simulink model "w3_warplab_trigger_proc"  (Simulink 7.7)
settings: Solver=ode45  StartTime=0.0  StopTime=60  RelTol=1e-3
InitFcn:
  | w3_warplab_trigger_proc_init
StartFcn:
  | w3_warplab_trigger_proc_init
undefined symbols (not defined in the file or in its folder): gcbh, xlBlockLoadCallback, xlGetNormalizedPeriod
libraries: xbsIndex_r4 x1289, xbsEDKLib_r4 x1, simulink x1
(part 1 of 10)
settings Model: Creator=murphpo  LastModifiedBy=mango
settings DebuggingCC: FcnCallInpInsideContextMsg=Enable All

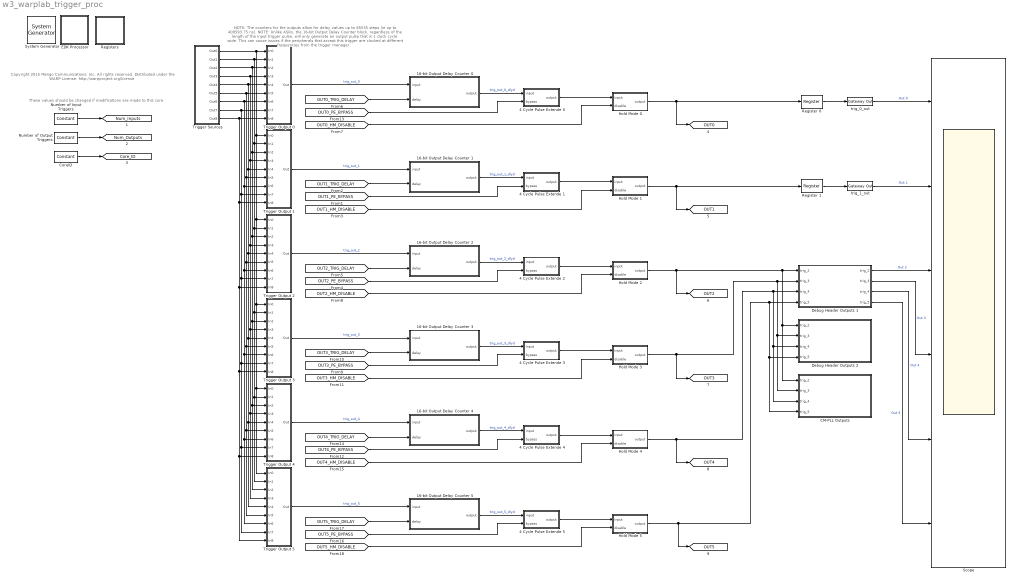
== system w3_warplab_trigger_proc ==
  note: These values should be changed if modifications are made to this core
  note: Copyright 2015 Mango Communications, Inc. All rights reserved.
      |
      | Distributed under the WARP License:
      | http://warpproject.org/license
  note: NOTE:  The counters for the outputs allow for delay values up to 65535 steps (ie up to 409593.75 ns).
      |
      | NOTE:  Unlike ASRs, the 16-bit Output Delay Counter block, regardless of the length of the input trigger
      | pulse, will only generate an output pulse that is 1 clock cycle wide. This can cause issues if the peripherals
      | that accept this trigger are clocked at different frequencies from the trigger manager.
  " System Generator" : xbsIndex_r4/ System Generator  Tag=genX  SystemSampleTime=-1  xilinxfamily=virtex6  part=xc6vlx240t  speed=-2  package=ff1156  synthesis_tool=XST  clock_wrapper=Clock Enables  directory=./trigger_proc  proj_type=Project Navigator  Synth_file=XST Defaults  Impl_file=ISE Defaults  testbench=off  simulink_period=1  sysclk_period=10  dcm_input_clock_period=10  incr_netlist=off  trim_vbits=Everywhere in SubSystem  dbl_ovrd=According to Block Masks  core_generation=According to Block Masks  run_coregen=off  deprecated_control=off  eval_field=0  block_type=sysgen
  16-bit Output Delay Counter 0 : Subsystem
  16-bit Output Delay Counter 1 : Subsystem
  16-bit Output Delay Counter 2 : Subsystem
  16-bit Output Delay Counter 3 : Subsystem
  16-bit Output Delay Counter 4 : Subsystem
  16-bit Output Delay Counter 5 : Subsystem
  4 Cycle Pulse Extende 0 : Subsystem
  4 Cycle Pulse Extende 1 : Subsystem
  4 Cycle Pulse Extende 2 : Subsystem
  4 Cycle Pulse Extende 3 : Subsystem
  4 Cycle Pulse Extende 4 : Subsystem
  4 Cycle Pulse Extende 5 : Subsystem
  CM-PLL Outputs : Subsystem
  CoreID : xbsIndex_r4/Constant  const=0  gui_display_data_type=Fixed-point  arith_type=Unsigned  n_bits=8  bin_pt=0  preci_type=Single  exp_width=8  frac_width=24  explicit_period=on  period=1  equ=P=C  opselect=C  inp2=PCIN>>17  opr=+  inp1=P  carry=CIN  dbl_ovrd=off  block_type=constant
  Debug Header Outputs 1 : Subsystem
  Debug Header Outputs 2 : Subsystem
  EDK Processor : Subsystem  LoadFcn=xlBlockLoadCallback(gcbh);  mask(Xilinx EDK Processor Block){mode=EDK pcore generation, xmp=, MemVisToProc=<qt bgcolor="#FFFFFF"><div><img src="C:/Xilinx/14.4/ISE_DS/ISE/sysgen/data/images/registerplus.gif"> &lt;&lt;TRIG_ODELAY_CFG_CMPLL&gt;&gt;<br></div><div><img src="C:/Xilinx/14.4/ISE_DS/ISE/sysgen/data/images/registerplus.gif"> &lt;&lt;TRIG_IDELAY_CFG_CMPLL&gt;&gt;<br></div><div><img src="C:/Xilinx/14.4/ISE_DS/ISE/sysgen/data/images/registerplus.gif"> &lt;&lt;TRIG_ODELAY_CFG_DEBUG_HDR&gt;&gt;<br></div><div><img src="C:/Xilinx/14.4/ISE_DS/ISE/sysgen/data/images/registerplus.gif"> &lt;&lt;TRIG_IDELAY_CFG_DEBUG_HDR&gt;&gt;<br></div><div><img src="C:/Xilinx/14.4/ISE_DS/ISE/sysgen/data/images/registerplus.gif"> &lt;&lt;TRIG_IODELAYS_CONTROL&gt;&gt;<br></div><div><img src="C:/Xilinx/14.4/ISE_DS/ISE/sysgen/data/images/registerplus.gif"> &lt;&lt;RSSI_PKT_DET_CONFIG&gt;&gt;<br></div><div><img src="C:/Xilinx/14.4/ISE_DS/ISE/sysgen/data/images/registerplus.gif"> &lt;&lt;TRIG_IN_CONF_6&gt;&gt;<br></div><div><img src="C:/Xilinx/14.4/ISE_DS/ISE/sysgen/data/images/registerplus.gif"> &lt;&lt;TRIG_IN_CONF_5&gt;&gt;<br></div><div><img src="C:/Xilinx/14.4/ISE_DS/ISE/sysgen/data/images/registerplus.gif"> &lt;&lt;TRIG_IN_CONF_4&gt;&gt;<br></div><div><img src="C:/Xilinx/14.4/ISE_DS/ISE/sysgen/data/images/registerplus.gif"> &lt;&lt;TRIG_IN_CONF_3&gt;&gt;<br></div><div><img src="C:/Xilinx/14.4/ISE_DS/ISE/sysgen/data/images/registerplus.gif"> &lt;&lt;TRIG_IN_CONF_2&gt;&gt;<br></div><div><img src="C:/Xilinx/14.4/ISE_DS/ISE/sysgen/data/images/registerplus.gif"> &lt;&lt;TRIG_IN_CONF_0&gt;&gt;<br></div><div><img src="C:/Xilinx/14.4/ISE_DS/ISE/sysgen/data/images/registerplus.gif"> &lt;&lt;TRIG_IN_CONF_8&gt;&gt;<br></div><div><img src="C:/Xilinx/14.4/ISE_DS/ISE/sysgen/data/images/registerplus.gif"> &lt;&lt;TRIG_IN_CONF_7&gt;&gt;<br></div><div><img src="C:/Xilinx/14.4/ISE_DS/ISE/sysgen/data/images/registerplus.gif"> &lt;&lt;TRIG_OUT_5_CONF_0&gt;&gt;<br></div><div><img src="C:/Xilinx/14.4/ISE_DS/ISE/sysgen/data/images/registerplus.gif"> &lt;&lt;TRIG_OUT_5_CONF_1&gt;&gt;<br></div><div><img src="C:/Xilinx/14.4/ISE_DS/ISE/sysgen/data/images/registerplus.gif"> &lt;&lt;TRIG_OUT_4_CONF_0&gt;&gt;<br></div><div><img src="C:/Xilinx/14.4/ISE_DS/ISE/sysgen/data/images/registerplus.gif"> &lt;&lt;TRIG_OUT_0_CONF_0&gt;&gt;<br></div><div><img src="C:/Xilinx/14.4/ISE_DS/ISE/sysgen/data/images/registerplus.gif"> &lt;&lt;TRIG_OUT_4_CONF_1&gt;&gt;<br></div><div><img src="C:/Xilinx/14.4/ISE_DS/ISE/sysgen/data/images/registerplus.gif"> &lt;&lt;TRIG_OUT_3_CONF_0&gt;&gt;<br></div><div><img src="C:/Xilinx/14.4/ISE_DS/ISE/sysgen/data/images/registerplus.gif"> &lt;&lt;TRIG_OUT_3_CONF_1&gt;&gt;<br></div><div><img src="C:/Xilinx/14.4/ISE_DS/ISE/sysgen/data/images/registerplus.gif"> &lt;&lt;TRIG_OUT_2_CONF_0&gt;&gt;<br></div><div><img src="C:/Xilinx/14.4/ISE_DS/ISE/sysgen/data/images/registerplus.gif"> &lt;&lt;TRIG_OUT_2_CONF_1&gt;&gt;<br></div><div><img src="C:/Xilinx/14.4/ISE_DS/ISE/sysgen/data/images/registerplus.gif"> &lt;&lt;TRIG_OUT_1_CONF_0&gt;&gt;<br></div><div><img src="C:/Xilinx/14.4/ISE_DS/ISE/sysgen/data/images/registerplus.gif"> &lt;&lt;TRIG_OUT_1_CONF_1&gt;&gt;<br></div><div><img src="C:/Xilinx/14.4/ISE_DS/ISE/sysgen/data/images/registerplus.gif"> &lt;&lt;TRIG_OUT_0_CONF_1&gt;&gt;<br></div><div><img src="C:/Xilinx/14.4/ISE_DS/ISE/sysgen/data/images/registerplus.gif"> &lt;&lt;RSSI_PKT_DET_DURATIONS&gt;&gt;<br></div><div><img src="C:/Xilinx/14.4/ISE_DS/ISE/sysgen/data/images/registerplus.gif"> &lt;&lt;RSSI_PKT_DET_THRESHOLDS&gt;&gt;<br></div><div><img src="C:/Xilinx/14.4/ISE_DS/ISE/sysgen/data/images/registerplus.gif"> &lt;&lt;TRIG_IN_CONF_1&gt;&gt;<br></div><div><img src="C:/Xilinx/14.4/ISE_DS/ISE/sysgen/data/images/registerplus.gif"> &lt;&lt;CORE_INFO&gt;&gt;<br></div><div><img src="C:/Xilinx/14.4/ISE_DS/ISE/sysgen/data/images/registerplus.gif"> &lt;&lt;TRIG_OUT&gt;&gt;<br></div><div><img src="C:/Xilinx/14.4/ISE_DS/ISE/sysgen/data/images/memoryplus.gif"> &lt;&lt;PktOps1&gt;&gt;<br></div><div><img src="C:/Xilinx/14.4/ISE_DS/ISE/sysgen/data/images/memoryplus.gif"> &lt;&lt;PktTemplate1&gt;&gt;<br></div><div><img src="C:/Xilinx/14.4/ISE_DS/ISE/sysgen/data/images/memoryplus.gif"> &lt;&lt;PktOps0&gt;&gt;<br></div><div><img src="C:/Xilinx/14.4/ISE_DS/ISE/sysgen/data/images/memoryplus.gif"> &lt;&lt;PktTemplate0&gt;&gt;<br></div></qt>, AvailableMemories=<empty>, portInterfaceTable={'exposed'=>[],'portdir'=>[],'portname'=>[],'shortname'=>[]}, bus_type_sgadvanced=, bus_type=AXI, baseaddr=0x80000000, baseaddr_lock_sgadvanced=, baseaddr_lock=off, dual_clock_sgadvanced=, dual_clock=on, reg_readback_sgadvanced=, reg_readback=on, ucf_file=, inheritDeviceType_sgadvanced=, inheritDeviceType=off, elf_file=, codebug_sgadvanced=, codebug=on, clock_name=plb, internalPortList={}, resetPolarity=0, memxtable={'mladdr'=>[0.00000000000000000,1.00000000000000000,2.00000000000000000,3.00000000000000000,4.00000000000000000,5.00000000000000000,6.00000000000000000,7.00000000000000000,8.00000000000000000,9.00000000000000000,10.00000000000000000,11.00000000000000000,12.00000000000000000,13.00000000000000000,14.00000000000000000,15.00000000000000000,16.00000000000000000,17.00000000000000000,18.00000000000000000,19.00000000000000000,20.00000000000000000,21.00000000000000000,22.00000000000000000,23.00000000000000000,24.00000000000000000,25.00000000000000000,26.00000000000000000,27.00000000000000000,28.00000000000000000,0.00000000000000000,1.00000000000000000,-1.00000000000000000,-1.00000000000000000,-1.00000000000000000,-1.00000000000000000],'mlist'=>['w3_warplab_trigger_proc/Registers/Trig IODELAY Config/From Register28','w3_warplab_trigger_proc/Registers/Trig IODELAY Config/From Register27','w3_warplab_trigger_proc/Registers/Trig IODELAY Config/From Register26','w3_warplab_trigger_proc/Registers/Trig IODELAY Config/From Register25','w3_warplab_trigger_proc/Registers/Trig IODELAY Config/From Register1','w3_warplab_trigger_proc/Registers/From Register9','w3_warplab_trigger_proc/Registers/From Register8','w3_warplab_trigger_proc/Registers/From Register7','w3_warplab_trigger_proc/Registers/From Register6','w3_warplab_trigger_proc/Registers/From Register5','w3_warplab_trigger_proc/Registers/From Register4','w3_warplab_trigger_proc/Registers/From Register3','w3_warplab_trigger_proc/Registers/From Register24','w3_warplab_trigger_proc/Registers/From Register23','w3_warplab_trigger_proc/Registers/From Register22','w3_warplab_trigger_proc/Registers/From Register21','w3_warplab_trigger_proc/Registers/From Register20','w3_warplab_trigger_proc/Registers/From Register2','w3_warplab_trigger_proc/Registers/From Register19','w3_warplab_trigger_proc/Registers/From Register18','w3_warplab_trigger_proc/Registers/From Register17','w3_warplab_trigger_proc/Registers/From Register16','w3_warplab_trigger_proc/Registers/From Register15','w3_warplab_trigger_proc/Registers/From Register14','w3_warplab_trigger_proc/Registers/From Register13','w3_warplab_trigger_proc/Registers/From Register12','w3_warplab_trigger_proc/Registers/From Register11','w3_warplab_trigger_proc/Registers/From Register10','w3_warplab_trigger_proc/Registers/From Register1','w3_warplab_trigger_proc/Registers/To Register1','w3_warplab_trigger_proc/Registers/To Register','w3_warplab_trigger_proc/Trigger Sources/Ethernet B/Pkt Comp/Word Comp 1/Shared Memory2','w3_warplab_trigger_proc/Trigger Sources/Ethernet B/Pkt Comp/Word Comp 1/Shared Memory1','w3_warplab_trigger_proc/Trigger Sources/Ethernet A/Pkt Comp/Word Comp 0/Shared Memory2','w3_warplab_trigger_proc/Trigger Sources/Ethernet A/Pkt Comp/Word Comp 0/Shared Memory1'],'mlname'=>['\\'TRIG_ODELAY_CFG_CMPLL\\'','\\'TRIG_IDELAY_CFG_CMPLL\\'','\\'TRIG_ODELAY_CFG_DEBUG_HDR\\'','\\'TRIG_IDELAY_CFG_DEBUG_HDR\\'','\\'TRIG_IODELAYS_CONTROL\\'','\\'RSSI_PKT_DET_CONFIG\\'','\\'TRIG_IN_CONF_6\\'','\\'TRIG_IN_CONF_5\\'','\\'TRIG_IN_CONF_4\\'','\\'TRIG_IN_CONF_3\\'','\\'TRIG_IN_CONF_2\\'','\\'TRIG_IN_CONF_0\\'','\\'TRIG_IN_CONF_8\\'','\\'TRIG_IN_CONF_7\\'','\\'TRIG_OUT_5_CONF_0\\'','\\'TRIG_OUT_5_CONF_1\\'','\\'TRIG_OUT_4_CONF_0\\'','\\'TRIG_OUT_0_CONF_0\\'','\\'TRIG_OUT_4_CONF_1\\'','\\'TRIG_OUT_3_CONF_0\\'','\\'TRIG_OUT_3_CONF_1\\'','\\'TRIG_OUT_2_CONF_0\\'','\\'TRIG_OUT_2_CONF_1\\'','\\'TRIG_OUT_1_CONF_0\\'','\\'TRIG_OUT_1_CONF_1\\'','\\'TRIG_OUT_0_CONF_1\\'','\\'RSSI_PKT_DET_DURATIONS\\'','\\'RSSI_PKT_DET_THRESHOLDS\\'','\\'TRIG_IN_CONF_1\\'','\\'CORE_INFO\\'','\\'TRIG_OUT\\'','\\'PktOps1\\'','\\'PktTemplate1\\'','\\'PktOps0\\'','\\'PktTemplate0\\''],'mlstate'=>[0.00000000000000000,0.00000000000000000,0.00000000000000000,0.00000000000000000,0.00000000000000000,0.00000000000000000,0.00000000000000000,0.00000000000000000,0.00000000000000000,0.00000000000000000,0.00000000000000000,0.00000000000000000,0.00000000000000000,0.00000000000000000,0.00000000000000000,0.00000000000000000,0.00000000000000000,0.00000000000000000,0.00000000000000000,0.00000000000000000,0.00000000000000000,0.00000000000000000,0.00000000000000000,0.00000000000000000,0.00000000000000000,0.00000000000000000,0.00000000000000000,0.00000000000000000,0.00000000000000000,0.00000000000000000,0.00000000000000000,0.00000000000000000,0.00000000000000000,0.00000000000000000,0.00000000000000000]}, procinfo={}, memmapdirty=off, blockname=, xpsintstyle=default, has_advanced_control=0, sggui_pos=-1,-1,-1,-1, block_type=edkprocessor, block_version=2.7, sg_icon_stat=62,64,-1,-1,white,blue,0,07734,right,,[ ],[ ], sg_mask_display=|, sg_list_contents={'table'=>{'AvailableMemories'=>'popup(<empty>)'}}, sg_blockgui_xml=}
      mask sg_mask_display=|
      | fprintf('','COMMENT: begin icon graphics');
      | patch([0 62 62 0 0 ],[0 0 64 64 0 ],[0.77 0.82 0.91 ]);
      | plot([0 62 62 0 0 ],[0 0 64 64 0 ]);
      | patch([13.2 24.76 32.76 40.76 48.76 32.76 21.2 13.2 ],[40.88 40.88 48.88 40.88 48.88 48.88 48.88 40.88 ],[1 1 1 ]);
      | patch([21.2 32.76 24.76 13.2 21.2 ],[32.88 32.88 40.88 40.88 32.88 ],[0.931 0.946 0.973 ]);
      | patch([13.2 24.76 32.76 21.2 13.2 ],[24.88 24.88 32.88 32.88 24.88 ],[1 1 1 ]);
      | patch([21.2 48.76 40.76 32.76 24.76 13.2 21.2 ],[16.88 16.88 24.88 16.88 24.88 24.88 16.88 ],[0.931 0.946 0.973 ]);
      | fprintf('','COMMENT: end icon graphics');
      | fprintf('','COMMENT: begin icon text');
      | fprintf('','COMMENT: end icon text');
      mask prompts: mode "Configure Processor for"; xmp "XPS Project"; MemVisToProc ""; AvailableMemories "Available Memories"; portInterfaceTable ""; bus_type_sgadvanced ""; bus_type "Bus Type"; baseaddr "Base Address"; baseaddr_lock_sgadvanced ""; baseaddr_lock "Lock"; dual_clock_sgadvanced ""; dual_clock "Dual Clocks"; reg_readback_sgadvanced ""; reg_readback "Register Read-Back"; ucf_file "Constraint File"; inheritDeviceType_sgadvanced ""; inheritDeviceType "Inherit Device Type"; elf_file "Initial Program"; codebug_sgadvanced ""; codebug "Enable Co-Debug with Xilinx SDK (Beta)"; clock_name ""; internalPortList ""; resetPolarity ""; memxtable ""; procinfo ""; memmapdirty ""; blockname ""; xpsintstyle ""; has_advanced_control ""; sggui_pos ""; block_type ""; block_version ""; sg_icon_stat ""; sg_mask_display ""; sg_list_contents ""; sg_blockgui_xml ""
      mask help: Xilinx EDK Processor
      mask init:
      | try
      |   tmp_gcb = gcb;
      |   tmp_gcbh = gcbh;
      |   if (strcmp('SysGenIndex',get_param(bdroot(tmp_gcbh),'tag')) && ~isempty(regexp(bdroot(tmp_gcb), '^xbs', 'once')))
      |     return;
      |   end;
      |   xlMungeMaskParams;
      | 
      |   block_type='edkprocessor';
      | 
      |   serialized_declarations = '{''block_type''=>''String''}';
      |   xledkprocessor_init();
      |   ptable_ = xlblockprep(get_param(tmp_gcb, 'MaskWSVariables'));
      |   try
      |     xlBlockMoveCallback(tmp_gcbh);
      |   catch 
      |      clear global xl_updateicon_recursion_guard;
      |   end;
      | catch
      |   global dbgsysgen;
      |   if(~isempty(dbgsysgen) && dbgsysgen)
      |     e = regexprep(lasterr, '\n', '\nError: ');
      |     disp(['Error: While running MaskInit code on block ' tmp_gcb ': ' e]);
      |     error(e);
      |   end
      | end
      settings: CopyFcn=xlProcBlockCopyCallback(gcbh);xlBlockMoveCallback(gcbh);  DeleteFcn=xlDestroyGui(gcbh);  ModelCloseFcn=xlDestroyGui(gcbh);  PreSaveFcn=xlBlockPreSaveCallback(gcbh);  PostSaveFcn=xlBlockPostSaveCallback(gcbh);  DestroyFcn=xlDestroyGui(gcbh);  OpenFcn=bh=gcbh;xlProcBlockCallbacks('populatesharedmemorylistbox',bh);xlOpenGui(bh, 'edkprocessor_gui.xml', @xlProcBlockEnablement, @xlProcBlockAction);  CloseFcn=xlDestroyGui(gcbh);  MoveFcn=xlBlockMoveCallback(gcbh);
      mask Help: eval('');xlDoc('-book','sysgen','-topic','EDK_Processor');
      mask StyleString: popup(EDK pcore generation|HDL netlisting),edit,edit,edit,edit,edit,popup(AXI|PLB),edit,edit,checkbox,edit,checkbox,edit,checkbox,edit,edit,checkbox,edit,edit,checkbox,edit,edit,edit,edit,edit,edit,edit,edit,edit,edit,edit,edit,edit,edit,edit,edit
      mask Display:
      | fprintf('','COMMENT: begin icon graphics');
      | patch([0 62 62 0 0 ],[0 0 64 64 0 ],[0.77 0.82 0.91 ]);
      | plot([0 62 62 0 0 ],[0 0 64 64 0 ]);
      | patch([13.2 24.76 32.76 40.76 48.76 32.76 21.2 13.2 ],[40.88 40.88 48.88 40.88 48.88 48.88 48.88 40.88 ],[1 1 1 ]);
      | patch([21.2 32.76 24.76 13.2 21.2 ],[32.88 32.88 40.88 40.88 32.88 ],[0.931 0.946 0.973 ]);
      | patch([13.2 24.76 32.76 21.2 13.2 ],[24.88 24.88 32.88 32.88 24.88 ],[1 1 1 ]);
      | patch([21.2 48.76 40.76 32.76 24.76 13.2 21.2 ],[16.88 16.88 24.88 16.88 24.88 24.88 16.88 ],[0.931 0.946 0.973 ]);
      | fprintf('','COMMENT: end icon graphics');
      | fprintf('','COMMENT: begin icon text');
      | disp('');
      | 
      | fprintf('','COMMENT: end icon text');
  Hold Mode 0 : Subsystem
  Hold Mode 1 : Subsystem
  Hold Mode 2 : Subsystem
  Hold Mode 3 : Subsystem
  Hold Mode 4 : Subsystem
  Hold Mode 5 : Subsystem
  Number of Input Triggers : xbsIndex_r4/Constant  const=9  gui_display_data_type=Fixed-point  arith_type=Unsigned  n_bits=8  bin_pt=0  preci_type=Single  exp_width=8  frac_width=24  explicit_period=on  period=1  equ=P=C  opselect=C  inp2=PCIN>>17  opr=+  inp1=P  carry=CIN  dbl_ovrd=off  block_type=constant
  Number of Output Triggers : xbsIndex_r4/Constant  const=6  gui_display_data_type=Fixed-point  arith_type=Unsigned  n_bits=8  bin_pt=0  preci_type=Single  exp_width=8  frac_width=24  explicit_period=on  period=1  equ=P=C  opselect=C  inp2=PCIN>>17  opr=+  inp1=P  carry=CIN  dbl_ovrd=off  block_type=constant
  Register 0 : xbsIndex_r4/Register  init=0  rst=off  en=off  dbl_ovrd=off  block_type=register
  Register 1 : xbsIndex_r4/Register  init=0  rst=off  en=off  dbl_ovrd=off  block_type=register
  Registers : Subsystem
  Scope : Scope  NumInputPorts=6
      settings: YMin=-5~-5~-5~-5~-5~-5  YMax=5~5~5~5~5~5
  Trigger Output 0 : Subsystem
  Trigger Output 1 : Subsystem
  Trigger Output 2 : Subsystem
  Trigger Output 3 : Subsystem
  Trigger Output 4 : Subsystem
  Trigger Output 5 : Subsystem
  Trigger Sources : Subsystem
  trig_0_out : xbsIndex_r4/Gateway Out  inherit_from_input=off  hdl_port=on  timing_constraint=None  locs_specified=off  LOCs={}  UseAsDAC=off  DACChannel='1'  block_type=gatewayout
  trig_1_out : xbsIndex_r4/Gateway Out  inherit_from_input=off  hdl_port=on  timing_constraint=None  locs_specified=off  LOCs={}  UseAsDAC=off  DACChannel='1'  block_type=gatewayout
  tag scope: Core_ID=global, Num_Inputs=global, Num_Outputs=global, OUT0=global, OUT1=global, OUT2=global, OUT3=global, OUT4=global, OUT5=global
  wires:
  Trigger Sources/1(Out0) -> Trigger Output 0/1(In0), Trigger Output 4/1(In0), Trigger Output 5/1(In0), Trigger Output 3/1(In0), Trigger Output 2/1(In0), Trigger Output 1/1(In0)
  Trigger Sources/2(Out1) -> Trigger Output 0/2(In1), Trigger Output 4/2(In1), Trigger Output 5/2(In1), Trigger Output 3/2(In1), Trigger Output 2/2(In1), Trigger Output 1/2(In1)
  Trigger Sources/3(Out2) -> Trigger Output 0/3(In2), Trigger Output 4/3(In2), Trigger Output 5/3(In2), Trigger Output 3/3(In2), Trigger Output 2/3(In2), Trigger Output 1/3(In2)
  Trigger Sources/4(Out3) -> Trigger Output 0/4(In3), Trigger Output 4/4(In3), Trigger Output 5/4(In3), Trigger Output 3/4(In3), Trigger Output 2/4(In3), Trigger Output 1/4(In3)
  Trigger Sources/5(Out4) -> Trigger Output 0/5(In4), Trigger Output 4/5(In4), Trigger Output 5/5(In4), Trigger Output 3/5(In4), Trigger Output 2/5(In4), Trigger Output 1/5(In4)
  Trigger Sources/6(Out5) -> Trigger Output 0/6(In5), Trigger Output 4/6(In5), Trigger Output 5/6(In5), Trigger Output 3/6(In5), Trigger Output 2/6(In5), Trigger Output 1/6(In5)
  Trigger Sources/7(Out6) -> Trigger Output 0/7(In6), Trigger Output 4/7(In6), Trigger Output 5/7(In6), Trigger Output 3/7(In6), Trigger Output 2/7(In6), Trigger Output 1/7(In6)
  Trigger Sources/8(Out7) -> Trigger Output 0/8(In7), Trigger Output 4/8(In7), Trigger Output 5/8(In7), Trigger Output 3/8(In7), Trigger Output 2/8(In7), Trigger Output 1/8(In7)
  Number of Input Triggers/1 -> [Num_Inputs]
  Number of Output Triggers/1 -> [Num_Outputs]
  CoreID/1 -> [Core_ID]
  trig_0_out/1 -> Scope/1  "Out 0"
  trig_1_out/1 -> Scope/2  "Out 1"
  Debug Header Outputs 1/1(trig_2) -> Scope/3  "Out 2"
  Debug Header Outputs 1/2(trig_3) -> Scope/4  "Out 3"
  Debug Header Outputs 1/4(trig_5) -> Scope/6  "Out 5"
  Trigger Sources/9(Out8) -> Trigger Output 0/9(In8), Trigger Output 4/9(In8), Trigger Output 5/9(In8), Trigger Output 3/9(In8), Trigger Output 2/9(In8), Trigger Output 1/9(In8)
  Register 0/1 -> trig_0_out/1
  Register 1/1 -> trig_1_out/1
  Debug Header Outputs 1/3(trig_4) -> Scope/5  "Out 4"
  Trigger Output 0/1(Out) -> 16-bit Output Delay Counter 0/1("input ")  "trig_out_0"
  [OUT0_TRIG_DELAY] -> 16-bit Output Delay Counter 0/2(delay)
  16-bit Output Delay Counter 0/1(output) -> 4 Cycle Pulse Extende 0/1("input ")  "trig_out_0_dlyd"
  [OUT0_PE_BYPASS] -> 4 Cycle Pulse Extende 0/2(bypass)
  Hold Mode 2/1(output) -> Debug Header Outputs 1/1("trig_2 "), Debug Header Outputs 2/1("trig_2 "), CM-PLL Outputs/1("trig_2 "), [OUT2]
  Hold Mode 3/1(output) -> Debug Header Outputs 1/2("trig_3 "), Debug Header Outputs 2/2("trig_3 "), CM-PLL Outputs/2("trig_3 "), [OUT3]
  Hold Mode 4/1(output) -> Debug Header Outputs 1/3("trig_4 "), Debug Header Outputs 2/3("trig_4 "), CM-PLL Outputs/3("trig_4 "), [OUT4]
  Hold Mode 5/1(output) -> Debug Header Outputs 1/4("trig_5 "), Debug Header Outputs 2/4("trig_5 "), CM-PLL Outputs/4("trig_5 "), [OUT5]
  4 Cycle Pulse Extende 0/1(output) -> Hold Mode 0/1("input ")
  [OUT0_HM_DISABLE] -> Hold Mode 0/2(disable)
  Hold Mode 0/1(output) -> Register 0/1, [OUT0]
  Trigger Output 1/1(Out) -> 16-bit Output Delay Counter 1/1("input ")  "trig_out_1"
  [OUT1_TRIG_DELAY] -> 16-bit Output Delay Counter 1/2(delay)
  16-bit Output Delay Counter 1/1(output) -> 4 Cycle Pulse Extende 1/1("input ")  "trig_out_1_dlyd"
  [OUT1_PE_BYPASS] -> 4 Cycle Pulse Extende 1/2(bypass)
  4 Cycle Pulse Extende 1/1(output) -> Hold Mode 1/1("input ")
  [OUT1_HM_DISABLE] -> Hold Mode 1/2(disable)
  Trigger Output 2/1(Out) -> 16-bit Output Delay Counter 2/1("input ")  "trig_out_2"
  [OUT2_TRIG_DELAY] -> 16-bit Output Delay Counter 2/2(delay)
  16-bit Output Delay Counter 2/1(output) -> 4 Cycle Pulse Extende 2/1("input ")  "trig_out_2_dlyd"
  [OUT2_PE_BYPASS] -> 4 Cycle Pulse Extende 2/2(bypass)
  4 Cycle Pulse Extende 2/1(output) -> Hold Mode 2/1("input ")
  [OUT2_HM_DISABLE] -> Hold Mode 2/2(disable)
  Trigger Output 3/1(Out) -> 16-bit Output Delay Counter 3/1("input ")  "trig_out_3"
  [OUT3_TRIG_DELAY] -> 16-bit Output Delay Counter 3/2(delay)
  16-bit Output Delay Counter 3/1(output) -> 4 Cycle Pulse Extende 3/1("input ")  "trig_out_3_dlyd"
  [OUT3_PE_BYPASS] -> 4 Cycle Pulse Extende 3/2(bypass)
  4 Cycle Pulse Extende 3/1(output) -> Hold Mode 3/1("input ")
  [OUT3_HM_DISABLE] -> Hold Mode 3/2(disable)
  Trigger Output 4/1(Out) -> 16-bit Output Delay Counter 4/1("input ")  "trig_out_4"
  [OUT4_TRIG_DELAY] -> 16-bit Output Delay Counter 4/2(delay)
  16-bit Output Delay Counter 4/1(output) -> 4 Cycle Pulse Extende 4/1("input ")  "trig_out_4_dlyd"
  [OUT4_PE_BYPASS] -> 4 Cycle Pulse Extende 4/2(bypass)
  4 Cycle Pulse Extende 4/1(output) -> Hold Mode 4/1("input ")
  [OUT4_HM_DISABLE] -> Hold Mode 4/2(disable)
  Trigger Output 5/1(Out) -> 16-bit Output Delay Counter 5/1("input ")  "trig_out_5"
  [OUT5_TRIG_DELAY] -> 16-bit Output Delay Counter 5/2(delay)
  16-bit Output Delay Counter 5/1(output) -> 4 Cycle Pulse Extende 5/1("input ")  "trig_out_5_dlyd"
  [OUT5_PE_BYPASS] -> 4 Cycle Pulse Extende 5/2(bypass)
  4 Cycle Pulse Extende 5/1(output) -> Hold Mode 5/1("input ")
  [OUT5_HM_DISABLE] -> Hold Mode 5/2(disable)
  Hold Mode 1/1(output) -> Register 1/1, [OUT1]

== system w3_warplab_trigger_proc/16-bit Output Delay Counter 0 ==
  note: 16-bit Delay Counter:
      |
      | NOTE:  The total delay through this counter is 1 clock cycle greater than "delay"
      |
      | NOTE:  This delay counter can only accept triggers greater than 'delay' clock cycles apart.
      |     Because the timeout_counter counter uses an S-R latch for its enable that is triggered by
      |     the rising edge of the input, unless the latch is reset (ie the timeout_counter == delay),
      |     then another rising edge on the input will not change the behavior of the output.
      |
      | Logic:
      |
      | if (delay == 0)
      |     output = rising_edge(input)
      | else
      |     output = rising_edge(timeout_counter == delay)
  "input " : Inport
  delay : Inport  Port=2
  Constant : xbsIndex_r4/Constant  const=0  gui_display_data_type=Fixed-point  arith_type=Unsigned  n_bits=16  bin_pt=0  preci_type=Single  exp_width=8  frac_width=24  explicit_period=off  period=1  equ=P=C  opselect=C  inp2=PCIN>>17  opr=+  inp1=P  carry=CIN  dbl_ovrd=off  block_type=constant
  Inverter : xbsIndex_r4/Inverter  en=off  latency=0  dbl_ovrd=off  block_type=inv
  Logical2 : xbsIndex_r4/Logical  logical_function=OR  inputs=2  en=off  latency=0  precision=Full  arith_type=Unsigned  n_bits=16  bin_pt=0  align_bp=on  dbl_ovrd=off  block_type=logical
  Logical3 : xbsIndex_r4/Logical  logical_function=AND  inputs=2  en=off  latency=0  precision=Full  arith_type=Unsigned  n_bits=16  bin_pt=0  align_bp=on  dbl_ovrd=off  block_type=logical
  Logical4 : xbsIndex_r4/Logical  logical_function=AND  inputs=2  en=off  latency=0  precision=Full  arith_type=Unsigned  n_bits=16  bin_pt=0  align_bp=on  dbl_ovrd=off  block_type=logical
  Posedge 0 : Subsystem
  Posedge 1 : Subsystem
  Register 0 : xbsIndex_r4/Register  init=0  rst=off  en=off  dbl_ovrd=off  block_type=register
  Relational1 : xbsIndex_r4/Relational  mode=a=b  en=off  latency=0  dbl_ovrd=off  block_type=relational
      settings: xl_area=[5 0 0 9 0 0 0]  block_version=VER_STRING_GOES_HERE
  Relational4 : xbsIndex_r4/Relational  mode=a=b  en=off  latency=0  dbl_ovrd=off  block_type=relational
      settings: xl_area=[5 0 0 9 0 0 0]  block_version=VER_STRING_GOES_HERE
  S-R Latch : Subsystem
  timeout_counter : xbsIndex_r4/Counter  cnt_type=Free Running  cnt_to=Inf  operation=Up  start_count=0  cnt_by_val=1  arith_type=Unsigned  n_bits=16  bin_pt=0  load_pin=off  rst=on  en=on  explicit_period=on  period=1  dbl_ovrd=off  use_behavioral_HDL=off  implementation=Fabric  use_rpm=off  block_type=counter
      settings: xl_area=[10 18 0 18 0 0 0]  block_version=VER_STRING_GOES_HERE
  output : Outport
  wires:
  S-R Latch/1(Q) -> timeout_counter/2
  timeout_counter/1 -> Relational4/1
  Relational4/1 -> timeout_counter/1, S-R Latch/2(R), Posedge 1/1(D)
  delay/1 -> Relational4/2, Relational1/1
  Posedge 0/1(Q) -> S-R Latch/1(S), Register 0/1
  Constant/1 -> Relational1/2
  Relational1/1 -> Logical4/1, Inverter/1
  Posedge 1/1(Q) -> Logical3/1
  Inverter/1 -> Logical3/2
  Logical3/1 -> Logical2/1
  "input "/1 -> Posedge 0/1(D)
  Logical2/1 -> output/1
  Logical4/1 -> Logical2/2
  Register 0/1 -> Logical4/2

== system w3_warplab_trigger_proc/16-bit Output Delay Counter 1 ==
  note: 16-bit Delay Counter:
      |
      | NOTE:  The total delay through this counter is 1 clock cycle greater than "delay"
      |
      | NOTE:  This delay counter can only accept triggers greater than 'delay' clock cycles apart.
      |     Because the timeout_counter counter uses an S-R latch for its enable that is triggered by
      |     the rising edge of the input, unless the latch is reset (ie the timeout_counter == delay),
      |     then another rising edge on the input will not change the behavior of the output.
      |
      | Logic:
      |
      | if (delay == 0)
      |     output = rising_edge(input)
      | else
      |     output = rising_edge(timeout_counter == delay)
  "input " : Inport
  delay : Inport  Port=2
  Constant : xbsIndex_r4/Constant  const=0  gui_display_data_type=Fixed-point  arith_type=Unsigned  n_bits=16  bin_pt=0  preci_type=Single  exp_width=8  frac_width=24  explicit_period=off  period=1  equ=P=C  opselect=C  inp2=PCIN>>17  opr=+  inp1=P  carry=CIN  dbl_ovrd=off  block_type=constant
  Inverter : xbsIndex_r4/Inverter  en=off  latency=0  dbl_ovrd=off  block_type=inv
  Logical2 : xbsIndex_r4/Logical  logical_function=OR  inputs=2  en=off  latency=0  precision=Full  arith_type=Unsigned  n_bits=16  bin_pt=0  align_bp=on  dbl_ovrd=off  block_type=logical
  Logical3 : xbsIndex_r4/Logical  logical_function=AND  inputs=2  en=off  latency=0  precision=Full  arith_type=Unsigned  n_bits=16  bin_pt=0  align_bp=on  dbl_ovrd=off  block_type=logical
  Logical4 : xbsIndex_r4/Logical  logical_function=AND  inputs=2  en=off  latency=0  precision=Full  arith_type=Unsigned  n_bits=16  bin_pt=0  align_bp=on  dbl_ovrd=off  block_type=logical
  Posedge 0 : Subsystem
  Posedge 1 : Subsystem
  Register 0 : xbsIndex_r4/Register  init=0  rst=off  en=off  dbl_ovrd=off  block_type=register
  Relational1 : xbsIndex_r4/Relational  mode=a=b  en=off  latency=0  dbl_ovrd=off  block_type=relational
      settings: xl_area=[5 0 0 9 0 0 0]  block_version=VER_STRING_GOES_HERE
  Relational4 : xbsIndex_r4/Relational  mode=a=b  en=off  latency=0  dbl_ovrd=off  block_type=relational
      settings: xl_area=[5 0 0 9 0 0 0]  block_version=VER_STRING_GOES_HERE
  S-R Latch : Subsystem
  timeout_counter : xbsIndex_r4/Counter  cnt_type=Free Running  cnt_to=Inf  operation=Up  start_count=0  cnt_by_val=1  arith_type=Unsigned  n_bits=16  bin_pt=0  load_pin=off  rst=on  en=on  explicit_period=on  period=1  dbl_ovrd=off  use_behavioral_HDL=off  implementation=Fabric  use_rpm=off  block_type=counter
      settings: xl_area=[10 18 0 18 0 0 0]  block_version=VER_STRING_GOES_HERE
  output : Outport
  wires:
  S-R Latch/1(Q) -> timeout_counter/2
  timeout_counter/1 -> Relational4/1
  Relational4/1 -> timeout_counter/1, S-R Latch/2(R), Posedge 1/1(D)
  delay/1 -> Relational4/2, Relational1/1
  Posedge 0/1(Q) -> S-R Latch/1(S), Register 0/1
  Constant/1 -> Relational1/2
  Relational1/1 -> Logical4/1, Inverter/1
  Posedge 1/1(Q) -> Logical3/1
  Inverter/1 -> Logical3/2
  Logical3/1 -> Logical2/1
  "input "/1 -> Posedge 0/1(D)
  Logical2/1 -> output/1
  Logical4/1 -> Logical2/2
  Register 0/1 -> Logical4/2

== system w3_warplab_trigger_proc/16-bit Output Delay Counter 2 ==
  note: 16-bit Delay Counter:
      |
      | NOTE:  The total delay through this counter is 1 clock cycle greater than "delay"
      |
      | NOTE:  This delay counter can only accept triggers greater than 'delay' clock cycles apart.
      |     Because the timeout_counter counter uses an S-R latch for its enable that is triggered by
      |     the rising edge of the input, unless the latch is reset (ie the timeout_counter == delay),
      |     then another rising edge on the input will not change the behavior of the output.
      |
      | Logic:
      |
      | if (delay == 0)
      |     output = rising_edge(input)
      | else
      |     output = rising_edge(timeout_counter == delay)
  "input " : Inport
  delay : Inport  Port=2
  Constant : xbsIndex_r4/Constant  const=0  gui_display_data_type=Fixed-point  arith_type=Unsigned  n_bits=16  bin_pt=0  preci_type=Single  exp_width=8  frac_width=24  explicit_period=off  period=1  equ=P=C  opselect=C  inp2=PCIN>>17  opr=+  inp1=P  carry=CIN  dbl_ovrd=off  block_type=constant
  Inverter : xbsIndex_r4/Inverter  en=off  latency=0  dbl_ovrd=off  block_type=inv
  Logical2 : xbsIndex_r4/Logical  logical_function=OR  inputs=2  en=off  latency=0  precision=Full  arith_type=Unsigned  n_bits=16  bin_pt=0  align_bp=on  dbl_ovrd=off  block_type=logical
  Logical3 : xbsIndex_r4/Logical  logical_function=AND  inputs=2  en=off  latency=0  precision=Full  arith_type=Unsigned  n_bits=16  bin_pt=0  align_bp=on  dbl_ovrd=off  block_type=logical
  Logical4 : xbsIndex_r4/Logical  logical_function=AND  inputs=2  en=off  latency=0  precision=Full  arith_type=Unsigned  n_bits=16  bin_pt=0  align_bp=on  dbl_ovrd=off  block_type=logical
  Posedge 0 : Subsystem
  Posedge 1 : Subsystem
  Register 0 : xbsIndex_r4/Register  init=0  rst=off  en=off  dbl_ovrd=off  block_type=register
  Relational1 : xbsIndex_r4/Relational  mode=a=b  en=off  latency=0  dbl_ovrd=off  block_type=relational
      settings: xl_area=[5 0 0 9 0 0 0]  block_version=VER_STRING_GOES_HERE
  Relational4 : xbsIndex_r4/Relational  mode=a=b  en=off  latency=0  dbl_ovrd=off  block_type=relational
      settings: xl_area=[5 0 0 9 0 0 0]  block_version=VER_STRING_GOES_HERE
  S-R Latch : Subsystem
  timeout_counter : xbsIndex_r4/Counter  cnt_type=Free Running  cnt_to=Inf  operation=Up  start_count=0  cnt_by_val=1  arith_type=Unsigned  n_bits=16  bin_pt=0  load_pin=off  rst=on  en=on  explicit_period=on  period=1  dbl_ovrd=off  use_behavioral_HDL=off  implementation=Fabric  use_rpm=off  block_type=counter
      settings: xl_area=[10 18 0 18 0 0 0]  block_version=VER_STRING_GOES_HERE
  output : Outport
  wires:
  S-R Latch/1(Q) -> timeout_counter/2
  timeout_counter/1 -> Relational4/1
  Relational4/1 -> timeout_counter/1, S-R Latch/2(R), Posedge 1/1(D)
  delay/1 -> Relational4/2, Relational1/1
  Posedge 0/1(Q) -> S-R Latch/1(S), Register 0/1
  Constant/1 -> Relational1/2
  Relational1/1 -> Logical4/1, Inverter/1
  Posedge 1/1(Q) -> Logical3/1
  Inverter/1 -> Logical3/2
  Logical3/1 -> Logical2/1
  "input "/1 -> Posedge 0/1(D)
  Logical2/1 -> output/1
  Logical4/1 -> Logical2/2
  Register 0/1 -> Logical4/2

== system w3_warplab_trigger_proc/16-bit Output Delay Counter 3 ==
  note: 16-bit Delay Counter:
      |
      | NOTE:  The total delay through this counter is 1 clock cycle greater than "delay"
      |
      | NOTE:  This delay counter can only accept triggers greater than 'delay' clock cycles apart.
      |     Because the timeout_counter counter uses an S-R latch for its enable that is triggered by
      |     the rising edge of the input, unless the latch is reset (ie the timeout_counter == delay),
      |     then another rising edge on the input will not change the behavior of the output.
      |
      | Logic:
      |
      | if (delay == 0)
      |     output = rising_edge(input)
      | else
      |     output = rising_edge(timeout_counter == delay)
  "input " : Inport
  delay : Inport  Port=2
  Constant : xbsIndex_r4/Constant  const=0  gui_display_data_type=Fixed-point  arith_type=Unsigned  n_bits=16  bin_pt=0  preci_type=Single  exp_width=8  frac_width=24  explicit_period=off  period=1  equ=P=C  opselect=C  inp2=PCIN>>17  opr=+  inp1=P  carry=CIN  dbl_ovrd=off  block_type=constant
  Inverter : xbsIndex_r4/Inverter  en=off  latency=0  dbl_ovrd=off  block_type=inv
  Logical2 : xbsIndex_r4/Logical  logical_function=OR  inputs=2  en=off  latency=0  precision=Full  arith_type=Unsigned  n_bits=16  bin_pt=0  align_bp=on  dbl_ovrd=off  block_type=logical
  Logical3 : xbsIndex_r4/Logical  logical_function=AND  inputs=2  en=off  latency=0  precision=Full  arith_type=Unsigned  n_bits=16  bin_pt=0  align_bp=on  dbl_ovrd=off  block_type=logical
  Logical4 : xbsIndex_r4/Logical  logical_function=AND  inputs=2  en=off  latency=0  precision=Full  arith_type=Unsigned  n_bits=16  bin_pt=0  align_bp=on  dbl_ovrd=off  block_type=logical
  Posedge 0 : Subsystem
  Posedge 1 : Subsystem
  Register 0 : xbsIndex_r4/Register  init=0  rst=off  en=off  dbl_ovrd=off  block_type=register
  Relational1 : xbsIndex_r4/Relational  mode=a=b  en=off  latency=0  dbl_ovrd=off  block_type=relational
      settings: xl_area=[5 0 0 9 0 0 0]  block_version=VER_STRING_GOES_HERE
  Relational4 : xbsIndex_r4/Relational  mode=a=b  en=off  latency=0  dbl_ovrd=off  block_type=relational
      settings: xl_area=[5 0 0 9 0 0 0]  block_version=VER_STRING_GOES_HERE
  S-R Latch : Subsystem
  timeout_counter : xbsIndex_r4/Counter  cnt_type=Free Running  cnt_to=Inf  operation=Up  start_count=0  cnt_by_val=1  arith_type=Unsigned  n_bits=16  bin_pt=0  load_pin=off  rst=on  en=on  explicit_period=on  period=1  dbl_ovrd=off  use_behavioral_HDL=off  implementation=Fabric  use_rpm=off  block_type=counter
      settings: xl_area=[10 18 0 18 0 0 0]  block_version=VER_STRING_GOES_HERE
  output : Outport
  wires:
  S-R Latch/1(Q) -> timeout_counter/2
  timeout_counter/1 -> Relational4/1
  Relational4/1 -> timeout_counter/1, S-R Latch/2(R), Posedge 1/1(D)
  delay/1 -> Relational4/2, Relational1/1
  Posedge 0/1(Q) -> S-R Latch/1(S), Register 0/1
  Constant/1 -> Relational1/2
  Relational1/1 -> Logical4/1, Inverter/1
  Posedge 1/1(Q) -> Logical3/1
  Inverter/1 -> Logical3/2
  Logical3/1 -> Logical2/1
  "input "/1 -> Posedge 0/1(D)
  Logical2/1 -> output/1
  Logical4/1 -> Logical2/2
  Register 0/1 -> Logical4/2

== system w3_warplab_trigger_proc/16-bit Output Delay Counter 4 ==
  note: 16-bit Delay Counter:
      |
      | NOTE:  The total delay through this counter is 1 clock cycle greater than "delay"
      |
      | NOTE:  This delay counter can only accept triggers greater than 'delay' clock cycles apart.
      |     Because the timeout_counter counter uses an S-R latch for its enable that is triggered by
      |     the rising edge of the input, unless the latch is reset (ie the timeout_counter == delay),
      |     then another rising edge on the input will not change the behavior of the output.
      |
      | Logic:
      |
      | if (delay == 0)
      |     output = rising_edge(input)
      | else
      |     output = rising_edge(timeout_counter == delay)
  "input " : Inport
  delay : Inport  Port=2
  Constant : xbsIndex_r4/Constant  const=0  gui_display_data_type=Fixed-point  arith_type=Unsigned  n_bits=16  bin_pt=0  preci_type=Single  exp_width=8  frac_width=24  explicit_period=off  period=1  equ=P=C  opselect=C  inp2=PCIN>>17  opr=+  inp1=P  carry=CIN  dbl_ovrd=off  block_type=constant
  Inverter : xbsIndex_r4/Inverter  en=off  latency=0  dbl_ovrd=off  block_type=inv
  Logical2 : xbsIndex_r4/Logical  logical_function=OR  inputs=2  en=off  latency=0  precision=Full  arith_type=Unsigned  n_bits=16  bin_pt=0  align_bp=on  dbl_ovrd=off  block_type=logical
  Logical3 : xbsIndex_r4/Logical  logical_function=AND  inputs=2  en=off  latency=0  precision=Full  arith_type=Unsigned  n_bits=16  bin_pt=0  align_bp=on  dbl_ovrd=off  block_type=logical
  Logical4 : xbsIndex_r4/Logical  logical_function=AND  inputs=2  en=off  latency=0  precision=Full  arith_type=Unsigned  n_bits=16  bin_pt=0  align_bp=on  dbl_ovrd=off  block_type=logical
  Posedge 0 : Subsystem
  Posedge 1 : Subsystem
  Register 0 : xbsIndex_r4/Register  init=0  rst=off  en=off  dbl_ovrd=off  block_type=register
  Relational1 : xbsIndex_r4/Relational  mode=a=b  en=off  latency=0  dbl_ovrd=off  block_type=relational
      settings: xl_area=[5 0 0 9 0 0 0]  block_version=VER_STRING_GOES_HERE
  Relational4 : xbsIndex_r4/Relational  mode=a=b  en=off  latency=0  dbl_ovrd=off  block_type=relational
      settings: xl_area=[5 0 0 9 0 0 0]  block_version=VER_STRING_GOES_HERE
  S-R Latch : Subsystem
  timeout_counter : xbsIndex_r4/Counter  cnt_type=Free Running  cnt_to=Inf  operation=Up  start_count=0  cnt_by_val=1  arith_type=Unsigned  n_bits=16  bin_pt=0  load_pin=off  rst=on  en=on  explicit_period=on  period=1  dbl_ovrd=off  use_behavioral_HDL=off  implementation=Fabric  use_rpm=off  block_type=counter
      settings: xl_area=[10 18 0 18 0 0 0]  block_version=VER_STRING_GOES_HERE
  output : Outport
  wires:
  S-R Latch/1(Q) -> timeout_counter/2
  timeout_counter/1 -> Relational4/1
  Relational4/1 -> timeout_counter/1, S-R Latch/2(R), Posedge 1/1(D)
  delay/1 -> Relational4/2, Relational1/1
  Posedge 0/1(Q) -> S-R Latch/1(S), Register 0/1
  Constant/1 -> Relational1/2
  Relational1/1 -> Logical4/1, Inverter/1
  Posedge 1/1(Q) -> Logical3/1
  Inverter/1 -> Logical3/2
  Logical3/1 -> Logical2/1
  "input "/1 -> Posedge 0/1(D)
  Logical2/1 -> output/1
  Logical4/1 -> Logical2/2
  Register 0/1 -> Logical4/2

== system w3_warplab_trigger_proc/16-bit Output Delay Counter 5 ==
  note: 16-bit Delay Counter:
      |
      | NOTE:  The total delay through this counter is 1 clock cycle greater than "delay"
      |
      | NOTE:  This delay counter can only accept triggers greater than 'delay' clock cycles apart.
      |     Because the timeout_counter counter uses an S-R latch for its enable that is triggered by
      |     the rising edge of the input, unless the latch is reset (ie the timeout_counter == delay),
      |     then another rising edge on the input will not change the behavior of the output.
      |
      | Logic:
      |
      | if (delay == 0)
      |     output = rising_edge(input)
      | else
      |     output = rising_edge(timeout_counter == delay)
  "input " : Inport
  delay : Inport  Port=2
  Constant : xbsIndex_r4/Constant  const=0  gui_display_data_type=Fixed-point  arith_type=Unsigned  n_bits=16  bin_pt=0  preci_type=Single  exp_width=8  frac_width=24  explicit_period=off  period=1  equ=P=C  opselect=C  inp2=PCIN>>17  opr=+  inp1=P  carry=CIN  dbl_ovrd=off  block_type=constant
  Inverter : xbsIndex_r4/Inverter  en=off  latency=0  dbl_ovrd=off  block_type=inv
  Logical2 : xbsIndex_r4/Logical  logical_function=OR  inputs=2  en=off  latency=0  precision=Full  arith_type=Unsigned  n_bits=16  bin_pt=0  align_bp=on  dbl_ovrd=off  block_type=logical
  Logical3 : xbsIndex_r4/Logical  logical_function=AND  inputs=2  en=off  latency=0  precision=Full  arith_type=Unsigned  n_bits=16  bin_pt=0  align_bp=on  dbl_ovrd=off  block_type=logical
  Logical4 : xbsIndex_r4/Logical  logical_function=AND  inputs=2  en=off  latency=0  precision=Full  arith_type=Unsigned  n_bits=16  bin_pt=0  align_bp=on  dbl_ovrd=off  block_type=logical
  Posedge 0 : Subsystem
  Posedge 1 : Subsystem
  Register 0 : xbsIndex_r4/Register  init=0  rst=off  en=off  dbl_ovrd=off  block_type=register
  Relational1 : xbsIndex_r4/Relational  mode=a=b  en=off  latency=0  dbl_ovrd=off  block_type=relational
      settings: xl_area=[5 0 0 9 0 0 0]  block_version=VER_STRING_GOES_HERE
  Relational4 : xbsIndex_r4/Relational  mode=a=b  en=off  latency=0  dbl_ovrd=off  block_type=relational
      settings: xl_area=[5 0 0 9 0 0 0]  block_version=VER_STRING_GOES_HERE
  S-R Latch : Subsystem
  timeout_counter : xbsIndex_r4/Counter  cnt_type=Free Running  cnt_to=Inf  operation=Up  start_count=0  cnt_by_val=1  arith_type=Unsigned  n_bits=16  bin_pt=0  load_pin=off  rst=on  en=on  explicit_period=on  period=1  dbl_ovrd=off  use_behavioral_HDL=off  implementation=Fabric  use_rpm=off  block_type=counter
      settings: xl_area=[10 18 0 18 0 0 0]  block_version=VER_STRING_GOES_HERE
  output : Outport
  wires:
  S-R Latch/1(Q) -> timeout_counter/2
  timeout_counter/1 -> Relational4/1
  Relational4/1 -> timeout_counter/1, S-R Latch/2(R), Posedge 1/1(D)
  delay/1 -> Relational4/2, Relational1/1
  Posedge 0/1(Q) -> S-R Latch/1(S), Register 0/1
  Constant/1 -> Relational1/2
  Relational1/1 -> Logical4/1, Inverter/1
  Posedge 1/1(Q) -> Logical3/1
  Inverter/1 -> Logical3/2
  Logical3/1 -> Logical2/1
  "input "/1 -> Posedge 0/1(D)
  Logical2/1 -> output/1
  Logical4/1 -> Logical2/2
  Register 0/1 -> Logical4/2

== system w3_warplab_trigger_proc/4 Cycle Pulse Extende 0 ==
  "input " : Inport
  bypass : Inport  Port=2
  Logical1 : xbsIndex_r4/Logical  logical_function=OR  inputs=4  en=off  latency=0  precision=Full  arith_type=Unsigned  n_bits=16  bin_pt=0  align_bp=on  dbl_ovrd=off  block_type=logical
      settings: xl_area=[1 0 0 1 0 0 0]  block_version=VER_STRING_GOES_HERE
  Mux : xbsIndex_r4/Mux  inputs=2  en=off  latency=0  precision=Full  arith_type=Unsigned  n_bits=16  bin_pt=14  quantization=Truncate  overflow=Wrap  dbl_ovrd=off  block_type=mux
  Register 1 : xbsIndex_r4/Register  init=0  rst=off  en=off  dbl_ovrd=off  block_type=register
  Register 2 : xbsIndex_r4/Register  init=0  rst=off  en=off  dbl_ovrd=off  block_type=register
  Register 3 : xbsIndex_r4/Register  init=0  rst=off  en=off  dbl_ovrd=off  block_type=register
  output : Outport
  wires:
  Mux/1 -> output/1
  "input "/1 -> Register 1/1, Logical1/1, Mux/3
  bypass/1 -> Mux/1
  Register 1/1 -> Register 2/1, Logical1/2
  Register 2/1 -> Register 3/1, Logical1/3
  Logical1/1 -> Mux/2
  Register 3/1 -> Logical1/4

== system w3_warplab_trigger_proc/4 Cycle Pulse Extende 1 ==
  "input " : Inport
  bypass : Inport  Port=2
  Logical1 : xbsIndex_r4/Logical  logical_function=OR  inputs=4  en=off  latency=0  precision=Full  arith_type=Unsigned  n_bits=16  bin_pt=0  align_bp=on  dbl_ovrd=off  block_type=logical
      settings: xl_area=[1 0 0 1 0 0 0]  block_version=VER_STRING_GOES_HERE
  Mux : xbsIndex_r4/Mux  inputs=2  en=off  latency=0  precision=Full  arith_type=Unsigned  n_bits=16  bin_pt=14  quantization=Truncate  overflow=Wrap  dbl_ovrd=off  block_type=mux
  Register 1 : xbsIndex_r4/Register  init=0  rst=off  en=off  dbl_ovrd=off  block_type=register
  Register 2 : xbsIndex_r4/Register  init=0  rst=off  en=off  dbl_ovrd=off  block_type=register
  Register 3 : xbsIndex_r4/Register  init=0  rst=off  en=off  dbl_ovrd=off  block_type=register
  output : Outport
  wires:
  Mux/1 -> output/1
  "input "/1 -> Register 1/1, Logical1/1, Mux/3
  bypass/1 -> Mux/1
  Register 1/1 -> Register 2/1, Logical1/2
  Register 2/1 -> Register 3/1, Logical1/3
  Logical1/1 -> Mux/2
  Register 3/1 -> Logical1/4

== system w3_warplab_trigger_proc/4 Cycle Pulse Extende 2 ==
  "input " : Inport
  bypass : Inport  Port=2
  Logical1 : xbsIndex_r4/Logical  logical_function=OR  inputs=4  en=off  latency=0  precision=Full  arith_type=Unsigned  n_bits=16  bin_pt=0  align_bp=on  dbl_ovrd=off  block_type=logical
      settings: xl_area=[1 0 0 1 0 0 0]  block_version=VER_STRING_GOES_HERE
  Mux : xbsIndex_r4/Mux  inputs=2  en=off  latency=0  precision=Full  arith_type=Unsigned  n_bits=16  bin_pt=14  quantization=Truncate  overflow=Wrap  dbl_ovrd=off  block_type=mux
  Register 1 : xbsIndex_r4/Register  init=0  rst=off  en=off  dbl_ovrd=off  block_type=register
  Register 2 : xbsIndex_r4/Register  init=0  rst=off  en=off  dbl_ovrd=off  block_type=register
  Register 3 : xbsIndex_r4/Register  init=0  rst=off  en=off  dbl_ovrd=off  block_type=register
  output : Outport
  wires:
  Mux/1 -> output/1
  "input "/1 -> Register 1/1, Logical1/1, Mux/3
  bypass/1 -> Mux/1
  Register 1/1 -> Register 2/1, Logical1/2
  Register 2/1 -> Register 3/1, Logical1/3
  Logical1/1 -> Mux/2
  Register 3/1 -> Logical1/4

== system w3_warplab_trigger_proc/4 Cycle Pulse Extende 3 ==
  "input " : Inport
  bypass : Inport  Port=2
  Logical1 : xbsIndex_r4/Logical  logical_function=OR  inputs=4  en=off  latency=0  precision=Full  arith_type=Unsigned  n_bits=16  bin_pt=0  align_bp=on  dbl_ovrd=off  block_type=logical
      settings: xl_area=[1 0 0 1 0 0 0]  block_version=VER_STRING_GOES_HERE
  Mux : xbsIndex_r4/Mux  inputs=2  en=off  latency=0  precision=Full  arith_type=Unsigned  n_bits=16  bin_pt=14  quantization=Truncate  overflow=Wrap  dbl_ovrd=off  block_type=mux
  Register 1 : xbsIndex_r4/Register  init=0  rst=off  en=off  dbl_ovrd=off  block_type=register
  Register 2 : xbsIndex_r4/Register  init=0  rst=off  en=off  dbl_ovrd=off  block_type=register
  Register 3 : xbsIndex_r4/Register  init=0  rst=off  en=off  dbl_ovrd=off  block_type=register
  output : Outport
  wires:
  Mux/1 -> output/1
  "input "/1 -> Register 1/1, Logical1/1, Mux/3
  bypass/1 -> Mux/1
  Register 1/1 -> Register 2/1, Logical1/2
  Register 2/1 -> Register 3/1, Logical1/3
  Logical1/1 -> Mux/2
  Register 3/1 -> Logical1/4

== system w3_warplab_trigger_proc/4 Cycle Pulse Extende 4 ==
  "input " : Inport
  bypass : Inport  Port=2
  Logical1 : xbsIndex_r4/Logical  logical_function=OR  inputs=4  en=off  latency=0  precision=Full  arith_type=Unsigned  n_bits=16  bin_pt=0  align_bp=on  dbl_ovrd=off  block_type=logical
      settings: xl_area=[1 0 0 1 0 0 0]  block_version=VER_STRING_GOES_HERE
  Mux : xbsIndex_r4/Mux  inputs=2  en=off  latency=0  precision=Full  arith_type=Unsigned  n_bits=16  bin_pt=14  quantization=Truncate  overflow=Wrap  dbl_ovrd=off  block_type=mux
  Register 1 : xbsIndex_r4/Register  init=0  rst=off  en=off  dbl_ovrd=off  block_type=register
  Register 2 : xbsIndex_r4/Register  init=0  rst=off  en=off  dbl_ovrd=off  block_type=register
  Register 3 : xbsIndex_r4/Register  init=0  rst=off  en=off  dbl_ovrd=off  block_type=register
  output : Outport
  wires:
  Mux/1 -> output/1
  "input "/1 -> Register 1/1, Logical1/1, Mux/3
  bypass/1 -> Mux/1
  Register 1/1 -> Register 2/1, Logical1/2
  Register 2/1 -> Register 3/1, Logical1/3
  Logical1/1 -> Mux/2
  Register 3/1 -> Logical1/4

== system w3_warplab_trigger_proc/4 Cycle Pulse Extende 5 ==
  "input " : Inport
  bypass : Inport  Port=2
  Logical1 : xbsIndex_r4/Logical  logical_function=OR  inputs=4  en=off  latency=0  precision=Full  arith_type=Unsigned  n_bits=16  bin_pt=0  align_bp=on  dbl_ovrd=off  block_type=logical
      settings: xl_area=[1 0 0 1 0 0 0]  block_version=VER_STRING_GOES_HERE
  Mux : xbsIndex_r4/Mux  inputs=2  en=off  latency=0  precision=Full  arith_type=Unsigned  n_bits=16  bin_pt=14  quantization=Truncate  overflow=Wrap  dbl_ovrd=off  block_type=mux
  Register 1 : xbsIndex_r4/Register  init=0  rst=off  en=off  dbl_ovrd=off  block_type=register
  Register 2 : xbsIndex_r4/Register  init=0  rst=off  en=off  dbl_ovrd=off  block_type=register
  Register 3 : xbsIndex_r4/Register  init=0  rst=off  en=off  dbl_ovrd=off  block_type=register
  output : Outport
  wires:
  Mux/1 -> output/1
  "input "/1 -> Register 1/1, Logical1/1, Mux/3
  bypass/1 -> Mux/1
  Register 1/1 -> Register 2/1, Logical1/2
  Register 2/1 -> Register 3/1, Logical1/3
  Logical1/1 -> Mux/2
  Register 3/1 -> Logical1/4
